simulink model "I2C_Master_Test"  (R2015b)
settings: Solver=FixedStepDiscrete  StartTime=0.0  StopTime=10.0  FixedStep=0.1  RelTol=1e-3
libraries: GPIO_Lib x8, I2C_Lib x4, STM32_Config_Lib x1
settings Model: Creator=liprandd  LastModifiedBy=reynaudp
settings DataIOCC: SaveFormat=Array
settings OptimizationCC: OptimizeModelRefInitCode=on  LifeSpan=1
settings DebuggingCC: UnderspecifiedInitializationDetection=Classic  MergeDetectMultiDrivingBlocksExec=none  SolverPrmCheckMsg=warning
settings HardwareCC: ProdBitPerPointer=32  ProdLargestAtomicInteger=Integer  ProdWordSize=32  ProdHWDeviceType=STMicroelectronics->STM32 32-bit Cortex-M
settings RTWCC: SystemTargetFile=stm32.tlc  TemplateMakefile=stm32.tmf  Description=stm32 (Embedded Target)  GenerateReport=on  IncludeHyperlinkInReport=on  LaunchReport=on
settings CodeAppCC: IgnoreCustomStorageClasses=off  MaxIdLength=64  CustomSymbolStrType=$N$R$M
settings STFCustomTargetCC: ParMdlRefBuildCompliant=on  ConcurrentExecutionCompliant=off  IncludeMdlTerminateFcn=off  GeneratePreprocessorConditionals=Use local settings  CombineOutputUpdateFcns=on  ERTCustomFileBanners=on  SupportContinuousTime=off  MATLABClassNameForMDSCustomization=Simulink.SoftwareTarget.ERTCustomization  CPPClassGenCompliant=off  GRTInterface=off  SystemTargetFile=stm32.tlc
settings ERTTargetCC: CompOptLevelCompliant=off  ConcurrentExecutionCompliant=off  IncludeMdlTerminateFcn=off  ERTFirstTimeCompliant=off  SupportNonInlinedSFcns=on  ModelStepFunctionPrototypeControlCompliant=off  CPPClassGenCompliant=off  UseToolchainInfoCompliant=off  ERTSrcFileBannerTemplate=sourceFileTemplate.cgt  ERTHdrFileBannerTemplate=sourceFileTemplate.cgt  ERTDataSrcFileTemplate=sourceFileTemplate.cgt  ERTDataHdrFileTemplate=sourceFileTemplate.cgt  ERTCustomFileTemplate=customRoutineProcess.tlc
settings ConfigComp: CovModelRefEnable=Off  CovSFcnEnable=off

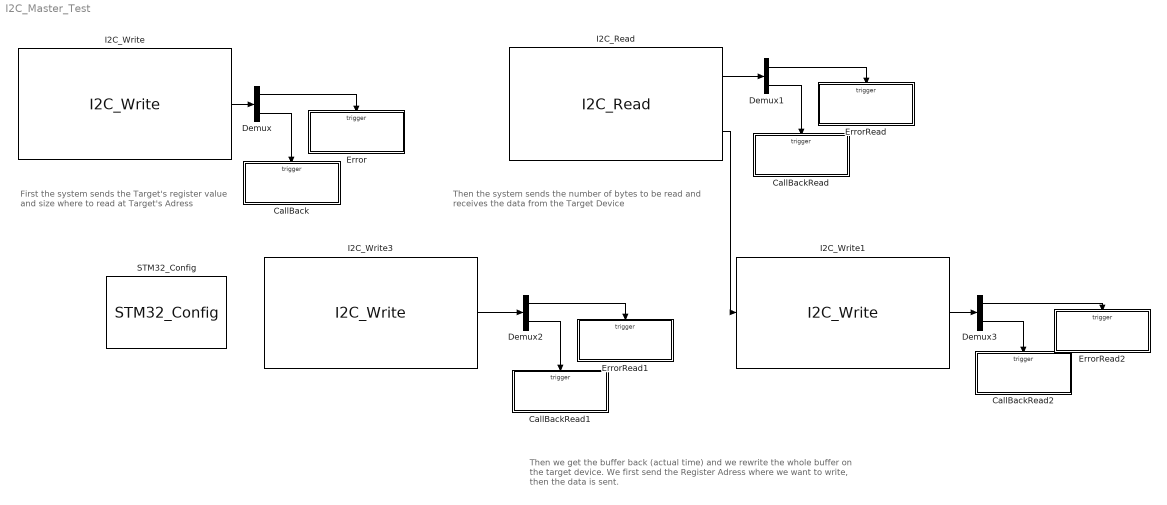
== system I2C_Master_Test ==
  note: First the system sends the
      | Target's register value and size
      | where to read at Target's Adress
  note: Then the system sends the
      | number of bytes to be read and
      | receives the data from the Target Device
  note: Then we get the buffer back (actual time)
      | and we rewrite the whole buffer on the target device.
      | We first send the Register Adress where we want to
      | write, then the data is sent.
  CallBack : Subsystem  TreatAsAtomicUnit=on
  CallBackRead : Subsystem  TreatAsAtomicUnit=on
  CallBackRead1 : Subsystem  TreatAsAtomicUnit=on
  CallBackRead2 : Subsystem  TreatAsAtomicUnit=on
  Demux{,1..3} (4 alike) : Demux  Outputs=2
  Error : Subsystem  TreatAsAtomicUnit=on
  ErrorRead : Subsystem  TreatAsAtomicUnit=on
  ErrorRead1 : Subsystem  TreatAsAtomicUnit=on
  ErrorRead2 : Subsystem  TreatAsAtomicUnit=on
  I2C_Read : I2C_Lib/I2C_Read  Priority=1  i2cx=I2C1  Device_Mode=MASTER  Device_Address=62  i2c_Mode=DMA_RX_TX  Target_Address=160  handler=hi2c1  Buffer_Size=3  Timeout=10  TimeoutValue=1  Enable_Output=on  Error=on  CallBack=on
  I2C_Write : I2C_Lib/I2C_Write  Priority=0  i2cx=I2C1  Device_Mode=MASTER  Target_Address=160  Target_Register=2  Enable_Input=off  Data_str={2}  i2c_Mode=DMA_RX_TX  Buffer_Size=1  handler=hi2c1  Timeout=10  TimeoutValue=1  Error=on  CallBack=on
  I2C_Write1 : I2C_Lib/I2C_Write  Priority=3  i2cx=I2C1  Device_Mode=MASTER  Target_Address=160  Target_Register=2  Enable_Input=on  Data_str_user=0x02,0x44,0x12  Data_str={2,0x02,0x44,0x12}  i2c_Mode=DMA_RX_TX  Buffer_Size=3  handler=hi2c1  Timeout=10  TimeoutValue=1  Error=on  CallBack=on
  I2C_Write3 : I2C_Lib/I2C_Write  Priority=2  i2cx=I2C1  Device_Mode=MASTER  Target_Address=160  Target_Register=2  Enable_Input=off  Data_str={2}  i2c_Mode=DMA_RX_TX  Buffer_Size=1  handler=hi2c1  Timeout=10  TimeoutValue=1  Error=on  CallBack=on
  STM32_Config : STM32_Config_Lib/STM32_Config  Project_Path=.\  Config_File=i2c_Master_Test.ioc  MCU_Name=STM32F429ZITx
  wires:
  I2C_Write/1 -> Demux/1
  Demux/2 -> CallBack/Trigger
  Demux/1 -> Error/Trigger
  I2C_Read/2 -> I2C_Write1/1
  I2C_Read/1 -> Demux1/1
  Demux1/2 -> CallBackRead/Trigger
  Demux1/1 -> ErrorRead/Trigger
  I2C_Write3/1 -> Demux2/1
  Demux2/2 -> CallBackRead1/Trigger
  Demux2/1 -> ErrorRead1/Trigger
  Demux3/2 -> CallBackRead2/Trigger
  Demux3/1 -> ErrorRead2/Trigger
  I2C_Write1/1 -> Demux3/1

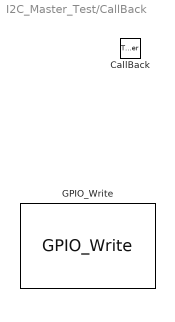
== system I2C_Master_Test/CallBack ==
  CallBack : TriggerPort  TriggerType=function-call
  GPIO_Write : GPIO_Lib/GPIO_Write  Port_name=GPIOE  Pin0=off  Toggle_Pin0=off  Pin1=off  Toggle_Pin1=off  Pin2=off  Toggle_Pin2=off  Pin3=off  Toggle_Pin3=off  Pin4=off  Toggle_Pin4=off  Pin5=off  Toggle_Pin5=off  Pin6=off  Toggle_Pin6=off  Pin7=off  Toggle_Pin7=off  Pin8=off  Toggle_Pin8=off  Pin9=on  Toggle_Pin9=on  Pin10=off  Toggle_Pin10=off  Pin11=off  Toggle_Pin11=off  Pin12=off  Toggle_Pin12=off  Pin13=off  Toggle_Pin13=off  Pin14=off  Toggle_Pin14=off  Pin15=off  Toggle_Pin15=off  PinList=GPIOA0GPIOE14

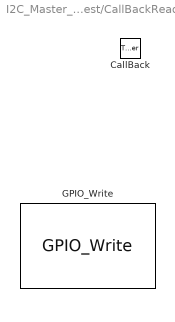
== system I2C_Master_Test/CallBackRead ==
  CallBack : TriggerPort  TriggerType=function-call
  GPIO_Write : GPIO_Lib/GPIO_Write  Port_name=GPIOE  Pin0=off  Toggle_Pin0=off  Pin1=off  Toggle_Pin1=off  Pin2=off  Toggle_Pin2=off  Pin3=off  Toggle_Pin3=off  Pin4=off  Toggle_Pin4=off  Pin5=off  Toggle_Pin5=off  Pin6=off  Toggle_Pin6=off  Pin7=off  Toggle_Pin7=off  Pin8=off  Toggle_Pin8=off  Pin9=off  Toggle_Pin9=off  Pin10=off  Toggle_Pin10=off  Pin11=on  Toggle_Pin11=on  Pin12=off  Toggle_Pin12=off  Pin13=off  Toggle_Pin13=off  Pin14=off  Toggle_Pin14=off  Pin15=off  Toggle_Pin15=off  PinList=GPIOA0GPIOE14

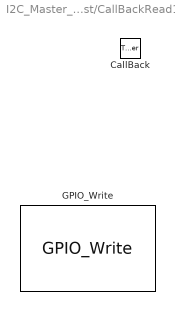
== system I2C_Master_Test/CallBackRead1 ==
  CallBack : TriggerPort  TriggerType=function-call
  GPIO_Write : GPIO_Lib/GPIO_Write  Port_name=GPIOE  Pin0=off  Toggle_Pin0=off  Pin1=off  Toggle_Pin1=off  Pin2=off  Toggle_Pin2=off  Pin3=off  Toggle_Pin3=off  Pin4=off  Toggle_Pin4=off  Pin5=off  Toggle_Pin5=off  Pin6=off  Toggle_Pin6=off  Pin7=off  Toggle_Pin7=off  Pin8=off  Toggle_Pin8=off  Pin9=off  Toggle_Pin9=off  Pin10=off  Toggle_Pin10=off  Pin11=off  Toggle_Pin11=off  Pin12=off  Toggle_Pin12=off  Pin13=on  Toggle_Pin13=on  Pin14=off  Toggle_Pin14=off  Pin15=off  Toggle_Pin15=off  PinList=GPIOA0GPIOE14

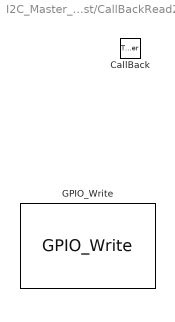
== system I2C_Master_Test/CallBackRead2 ==
  CallBack : TriggerPort  TriggerType=function-call
  GPIO_Write : GPIO_Lib/GPIO_Write  Port_name=GPIOE  Pin0=off  Toggle_Pin0=off  Pin1=off  Toggle_Pin1=off  Pin2=off  Toggle_Pin2=off  Pin3=off  Toggle_Pin3=off  Pin4=off  Toggle_Pin4=off  Pin5=off  Toggle_Pin5=off  Pin6=off  Toggle_Pin6=off  Pin7=off  Toggle_Pin7=off  Pin8=off  Toggle_Pin8=off  Pin9=off  Toggle_Pin9=off  Pin10=off  Toggle_Pin10=off  Pin11=off  Toggle_Pin11=off  Pin12=off  Toggle_Pin12=off  Pin13=off  Toggle_Pin13=off  Pin14=off  Toggle_Pin14=off  Pin15=on  Toggle_Pin15=on  PinList=GPIOA0GPIOE14

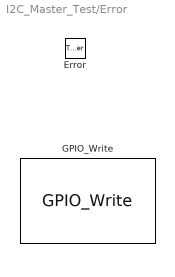
== system I2C_Master_Test/Error ==
  Error : TriggerPort  TriggerType=function-call
  GPIO_Write : GPIO_Lib/GPIO_Write  Port_name=GPIOE  Pin0=off  Toggle_Pin0=off  Pin1=off  Toggle_Pin1=off  Pin2=off  Toggle_Pin2=off  Pin3=off  Toggle_Pin3=off  Pin4=off  Toggle_Pin4=off  Pin5=off  Toggle_Pin5=off  Pin6=off  Toggle_Pin6=off  Pin7=off  Toggle_Pin7=off  Pin8=on  Toggle_Pin8=on  Pin9=off  Toggle_Pin9=off  Pin10=off  Toggle_Pin10=off  Pin11=off  Toggle_Pin11=off  Pin12=off  Toggle_Pin12=off  Pin13=off  Toggle_Pin13=off  Pin14=off  Toggle_Pin14=off  Pin15=off  Toggle_Pin15=off  PinList=GPIOA0GPIOE14

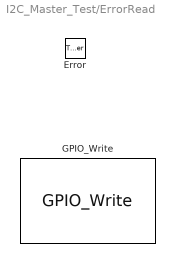
== system I2C_Master_Test/ErrorRead ==
  Error : TriggerPort  TriggerType=function-call
  GPIO_Write : GPIO_Lib/GPIO_Write  Port_name=GPIOE  Pin0=off  Toggle_Pin0=off  Pin1=off  Toggle_Pin1=off  Pin2=off  Toggle_Pin2=off  Pin3=off  Toggle_Pin3=off  Pin4=off  Toggle_Pin4=off  Pin5=off  Toggle_Pin5=off  Pin6=off  Toggle_Pin6=off  Pin7=off  Toggle_Pin7=off  Pin8=off  Toggle_Pin8=off  Pin9=off  Toggle_Pin9=off  Pin10=on  Toggle_Pin10=on  Pin11=off  Toggle_Pin11=off  Pin12=off  Toggle_Pin12=off  Pin13=off  Toggle_Pin13=off  Pin14=off  Toggle_Pin14=off  Pin15=off  Toggle_Pin15=off  PinList=GPIOA0GPIOE14

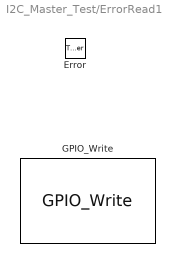
== system I2C_Master_Test/ErrorRead1 ==
  Error : TriggerPort  TriggerType=function-call
  GPIO_Write : GPIO_Lib/GPIO_Write  Port_name=GPIOE  Pin0=off  Toggle_Pin0=off  Pin1=off  Toggle_Pin1=off  Pin2=off  Toggle_Pin2=off  Pin3=off  Toggle_Pin3=off  Pin4=off  Toggle_Pin4=off  Pin5=off  Toggle_Pin5=off  Pin6=off  Toggle_Pin6=off  Pin7=off  Toggle_Pin7=off  Pin8=off  Toggle_Pin8=off  Pin9=off  Toggle_Pin9=off  Pin10=off  Toggle_Pin10=off  Pin11=off  Toggle_Pin11=off  Pin12=on  Toggle_Pin12=on  Pin13=off  Toggle_Pin13=off  Pin14=off  Toggle_Pin14=off  Pin15=off  Toggle_Pin15=off  PinList=GPIOA0GPIOE14

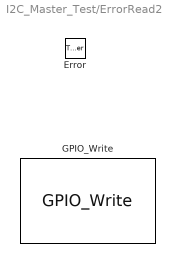
== system I2C_Master_Test/ErrorRead2 ==
  Error : TriggerPort  TriggerType=function-call
  GPIO_Write : GPIO_Lib/GPIO_Write  Port_name=GPIOE  Pin0=off  Toggle_Pin0=off  Pin1=off  Toggle_Pin1=off  Pin2=off  Toggle_Pin2=off  Pin3=off  Toggle_Pin3=off  Pin4=off  Toggle_Pin4=off  Pin5=off  Toggle_Pin5=off  Pin6=off  Toggle_Pin6=off  Pin7=off  Toggle_Pin7=off  Pin8=off  Toggle_Pin8=off  Pin9=off  Toggle_Pin9=off  Pin10=off  Toggle_Pin10=off  Pin11=off  Toggle_Pin11=off  Pin12=off  Toggle_Pin12=off  Pin13=off  Toggle_Pin13=off  Pin14=on  Toggle_Pin14=on  Pin15=off  Toggle_Pin15=off  PinList=GPIOA0GPIOE14
